simulink model "gm_sampleModel1607_1_sub"  (R2023a)
settings: Solver=VariableStepAuto  StartTime=0.0  StopTime=10.0  RelTol=1e-3
libraries: simulink x1, hdlsllib x1
settings Model: Creator=user1  LastModifiedBy=user1
settings OptimizationCC: BlockReduction=off  ConditionallyExecuteInputs=off
settings DebuggingCC: InheritedTsInSrcMsg=none

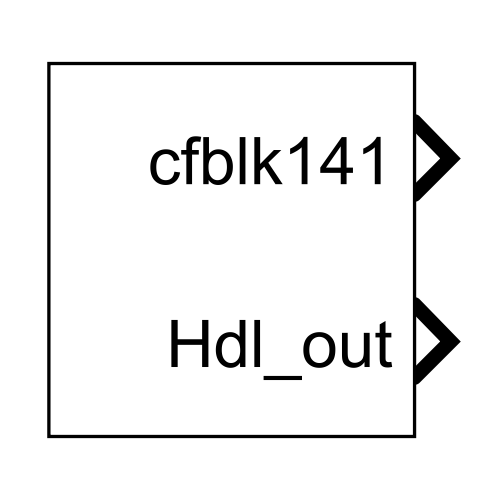
[thumbnail: Simulink's stored preview of the top-level diagram]
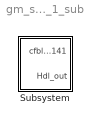
== system gm_sampleModel1607_1_sub ==
  Subsystem : Subsystem

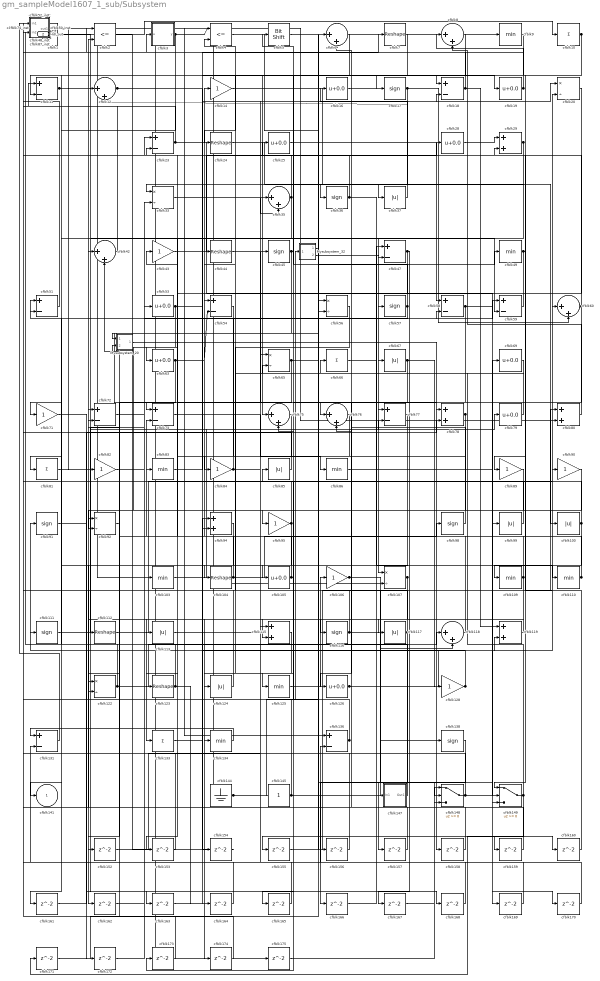
== system gm_sampleModel1607_1_sub/Subsystem ==
  Mysubsystem_20 : Subsystem
  Mysubsystem_32 : Subsystem
  cfblk1 : simulink/Logic and Bit Operations/Extract Bits  bitsToExtract=Upper half  numBits=8  bitIdxRange=[0 7]  outScalingMode=Preserve fixed-point scaling
      settings: LibrarySourceBlock=|
      | hdlsllib/Logic and Bit
      | Operations/Extract Bits
  cfblk{10,66,81,133} (4 alike) : Sum  Inputs=+  OutDataTypeStr=uint8
  cfblk{37,67,85,99..100,113,117,124} (8 alike) : Abs  OutDataTypeStr=uint8  SaturateOnIntegerOverflow=off
  cfblk101_inst : Subsystem
  cfblk{9,49,83,86,103,109..110,125,134} (9 alike) : MinMax  OutDataTypeStr=uint8
  cfblk{7,24,44,104,112,123} (6 alike) : Reshape
  cfblk{16,19,25,28,53,63,69,79,105,126} (10 alike) : Bias  Bias=0.0  SaturateOnIntegerOverflow=off
  cfblk{14,43,71,82,84,89..90,95,106,128} (10 alike) : Gain  OutDataTypeStr=uint8
  cfblk{20,33,56,65,92,107,122} (7 alike) : Product  Inputs=*/  OutDataTypeStr=uint8  RndMeth=Zero  SaturateOnIntegerOverflow=on
  cfblk{11,18,23,47,51,54,58..59,72..73,77,131,136} (13 alike) : Sum  Inputs=+-  OutDataTypeStr=uint8
  cfblk{17,36,45,57,91,98,111,116,138} (9 alike) : Signum
  cfblk{29,78,80,94,115,119} (6 alike) : Sum  OutDataTypeStr=uint8
  cfblk{6,8,12,35,42,60,75..76,118} (9 alike) : Sum  Inputs=|++  OutDataTypeStr=uint8
  cfblk130_inst : Subsystem
  cfblk144 : Ground
  cfblk145 : Constant  OutDataTypeStr=uint8  SampleTime=-1
  cfblk147 : Subsystem
  cfblk148 : Switch  OutDataTypeStr=uint8  SaturateOnIntegerOverflow=off  InputSameDT=off
  cfblk149 : Switch  OutDataTypeStr=uint8  SaturateOnIntegerOverflow=off  InputSameDT=off
  cfblk{152..175} (24 alike) : Delay  SampleTime=1
  cfblk15_inst : Subsystem
  cfblk2 : RelationalOperator  Operator=<=  OutDataTypeStr=boolean  InputSameDT=off
  cfblk3 : Subsystem  mask(Compare To Zero){relop=<=, OutDataTypeStr=uint8, ZeroCross=on}
      mask prompts: relop "Simulink:masks:Operator_MP"; OutDataTypeStr "Simulink:masks:OutputDataType_MP"; ZeroCross "Simulink:masks:EnableZerocrossingDetection_MP"
      mask help: Simulink:masks:CompareToZero_MD
      mask init:
      | OutDataTypeStr = 'uint8';
      | ZeroCross = 'on';
      | blkName = 'sampleModel1607_1_sub/Subsystem/cfblk3';
      | relop = '<=';
      | setValue = 'fixdt(0, 8)';
      mask TypeOptions relop: == | ~= | < | <= | >= | >
      mask TypeOptions OutDataTypeStr: Simulink:masks:uint8 | Simulink:masks:boolean
      mask Callback ZeroCross: sl('zeroCrossEnable', gcbh);
      mask Display: disp([relop,' 0'])
  cfblk4 : RelationalOperator  Operator=<=  OutDataTypeStr=boolean  InputSameDT=off
  cfblk48_inst : Subsystem
  cfblk5 : hdlsllib/Logic and Bit Operations/Bit Shift  mode=Shift Left Logical  N=0
  cfblk50_inst : Subsystem
  cfblk52_inst : Subsystem
  cfblk74_inst : Subsystem
  cfblk87_inst : Subsystem
  cfblk141 : Outport  OutDataTypeStr=uint8  SampleTime=1  VectorParamsAs1DForOutWhenUnconnected=off
  Hdl_out : Outport  Port=2  OutDataTypeStr=uint8  SampleTime=1
  wires:
  Mysubsystem_20/1(Out1) -> cfblk158/1
  Mysubsystem_32/1(Out1) -> cfblk73/1
  Mysubsystem_32/2(Out2) -> cfblk107/1
  cfblk1/1 -> cfblk59/2
  cfblk10/1 -> cfblk75/1, cfblk149/1
  cfblk100/1 -> cfblk23/2, cfblk109/1
  cfblk101_inst/1(out1) -> cfblk175/1
  cfblk103/1 -> cfblk77/2
  cfblk104/1 -> cfblk98/1, cfblk73/2
  cfblk105/1 -> cfblk173/1, cfblk14/1
  cfblk106/1 -> cfblk138/1, cfblk118/2
  cfblk107/1 -> cfblk174/1, cfblk133/1
  cfblk109/1 -> cfblk43/1, cfblk162/1
  cfblk11/1 -> cfblk47/2, cfblk168/1
  cfblk110/1 -> cfblk54/1, cfblk83/1
  cfblk111/1 -> cfblk79/1
  cfblk112/1 -> cfblk69/1
  cfblk113/1 -> cfblk45/1
  cfblk115/1 -> cfblk134/1
  cfblk116/1 -> cfblk2/2, cfblk149/3
  cfblk117/1 -> cfblk4/2, cfblk157/1
  cfblk118/1 -> Mysubsystem_20/2(In2)
  cfblk119/1 -> cfblk115/2
  cfblk12/1 -> cfblk18/1, cfblk154/1
  cfblk122/1 -> cfblk50_inst/2(in2), cfblk118/1
  cfblk123/1 -> cfblk91/1, cfblk164/1
  cfblk124/1 -> cfblk48_inst/2(in2)
  cfblk125/1 -> cfblk106/1
  cfblk126/1 -> cfblk99/1, cfblk20/2
  cfblk128/1 -> cfblk6/2, cfblk111/1
  cfblk130_inst/1(out1) -> cfblk17/1
  cfblk131/1 -> cfblk52_inst/1(in1)
  cfblk133/1 -> cfblk94/1
  cfblk134/1 -> cfblk131/1
  cfblk136/1 -> cfblk85/1, cfblk72/1
  cfblk138/1 -> cfblk166/1
  cfblk14/1 -> cfblk37/1
  cfblk144/1 -> cfblk6/1, Mysubsystem_32/1(In1)
  cfblk145/1 -> cfblk60/1, cfblk149/2, cfblk101_inst/2(in2)
  cfblk147/1(Out1) -> cfblk51/1
  cfblk148/1 -> cfblk52_inst/2(in2), cfblk90/1
  cfblk149/1 -> cfblk171/1, cfblk66/1
  cfblk15_inst/1(out1) -> cfblk107/2, cfblk147/1(In1)
  cfblk152/1 -> cfblk35/1
  cfblk153/1 -> cfblk50_inst/1(in1)
  cfblk154/1 -> cfblk1/1
  cfblk155/1 -> cfblk80/1
  cfblk156/1 -> cfblk42/2
  cfblk157/1 -> cfblk122/2
  cfblk158/1 -> cfblk74_inst/1(in1)
  cfblk159/1 -> cfblk76/2
  cfblk16/1 -> cfblk19/1
  cfblk160/1 -> cfblk29/2
  cfblk161/1 -> cfblk78/2
  cfblk162/1 -> cfblk33/2
  cfblk163/1 -> cfblk119/2
  cfblk164/1 -> cfblk131/2
  cfblk165/1 -> cfblk115/1
  cfblk166/1 -> cfblk47/1
  cfblk167/1 -> cfblk148/3
  cfblk168/1 -> cfblk15_inst/1(in1)
  cfblk169/1 -> cfblk136/2
  cfblk17/1 -> cfblk60/2, cfblk12/2, cfblk33/1
  cfblk170/1 -> cfblk87_inst/1(in1)
  cfblk171/1 -> cfblk56/2
  cfblk172/1 -> cfblk59/1
  cfblk173/1 -> cfblk72/2
  cfblk174/1 -> cfblk130_inst/2(in2)
  cfblk175/1 -> cfblk148/1
  cfblk18/1 -> cfblk87_inst/2(in2), cfblk119/1
  cfblk19/1 -> cfblk8/1, cfblk11/2, cfblk3/1(u)
  cfblk2/1 -> cfblk10/1
  cfblk20/1 -> cfblk105/1
  cfblk23/1 -> cfblk11/1, cfblk169/1
  cfblk24/1 -> cfblk100/1
  cfblk25/1 -> cfblk58/1
  cfblk28/1 -> cfblk29/1
  cfblk29/1 -> cfblk36/1, cfblk161/1
  cfblk3/1(y) -> cfblk4/1, cfblk71/1
  cfblk33/1 -> cfblk35/2
  cfblk35/1 -> cfblk63/1, cfblk15_inst/2(in2)
  cfblk36/1 -> cfblk25/1, cfblk110/1
  cfblk37/1 -> cfblk16/1
  cfblk4/1 -> cfblk156/1
  cfblk42/1 -> cfblk130_inst/1(in1)
  cfblk43/1 -> cfblk28/1
  cfblk44/1 -> cfblk77/1
  cfblk45/1 -> cfblk159/1, Mysubsystem_20/1(In1)
  cfblk47/1 -> cfblk67/1, cfblk123/1, cfblk167/1
  cfblk48_inst/1(out1) -> Hdl_out/1, cfblk103/1
  cfblk49/1 -> cfblk117/1, cfblk89/1
  cfblk5/1 -> cfblk148/2
  cfblk50_inst/1(out1) -> cfblk136/1
  cfblk51/1 -> cfblk74_inst/2(in2)
  cfblk52_inst/1(out1) -> cfblk80/2
  cfblk53/1 -> cfblk92/2, cfblk20/1
  cfblk54/1 -> cfblk153/1
  cfblk56/1 -> cfblk104/1
  cfblk57/1 -> cfblk51/2, cfblk5/1
  cfblk58/1 -> cfblk76/1, cfblk160/1
  cfblk59/1 -> cfblk57/1
  cfblk6/1 -> cfblk165/1
  cfblk60/1 -> cfblk23/1, cfblk126/1
  cfblk63/1 -> cfblk54/2, cfblk92/1
  cfblk65/1 -> cfblk113/1, cfblk49/1
  cfblk66/1 -> cfblk58/2
  cfblk67/1 -> cfblk128/1, cfblk125/1
  cfblk69/1 -> cfblk65/2
  cfblk7/1 -> cfblk75/2
  cfblk71/1 -> cfblk172/1
  cfblk72/1 -> cfblk78/1
  cfblk73/1 -> cfblk86/1
  cfblk74_inst/1(out1) -> cfblk12/1
  cfblk75/1 -> cfblk124/1
  cfblk76/1 -> cfblk94/2
  cfblk77/1 -> cfblk155/1
  cfblk78/1 -> cfblk116/1, cfblk84/1
  cfblk79/1 -> cfblk44/1
  cfblk8/1 -> cfblk24/1
  cfblk80/1 -> cfblk8/2
  cfblk81/1 -> cfblk53/1
  cfblk82/1 -> cfblk56/1
  cfblk83/1 -> cfblk7/1
  cfblk84/1 -> cfblk42/1, cfblk18/2
  cfblk85/1 -> cfblk101_inst/1(in1)
  cfblk86/1 -> cfblk170/1
  cfblk87_inst/1(out1) -> cfblk82/1, cfblk9/1
  cfblk89/1 -> cfblk95/1
  cfblk9/1 -> cfblk81/1
  cfblk90/1 -> cfblk122/1
  cfblk91/1 -> cfblk163/1
  cfblk92/1 -> cfblk152/1
  cfblk94/1 -> cfblk112/1
  cfblk95/1 -> cfblk48_inst/1(in1), cfblk141/1
  cfblk98/1 -> cfblk2/1
  cfblk99/1 -> cfblk65/1

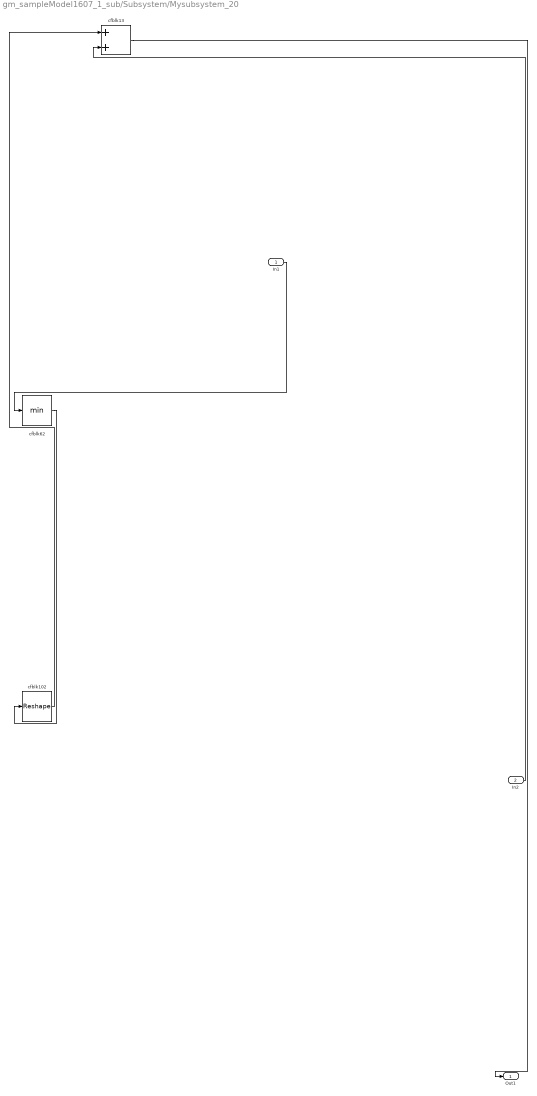
== system gm_sampleModel1607_1_sub/Subsystem/Mysubsystem_20 ==
  In1 : Inport  OutDataTypeStr=uint8  PortDimensions=1  SampleTime=1
  In2 : Inport  Port=2  OutDataTypeStr=uint8  PortDimensions=1  SampleTime=1
  cfblk102 : Reshape
  cfblk13 : Sum
  cfblk62 : MinMax
  Out1 : Outport  SampleTime=1
  wires:
  In1/1 -> cfblk62/1
  In2/1 -> cfblk13/2
  cfblk102/1 -> cfblk13/1
  cfblk13/1 -> Out1/1
  cfblk62/1 -> cfblk102/1

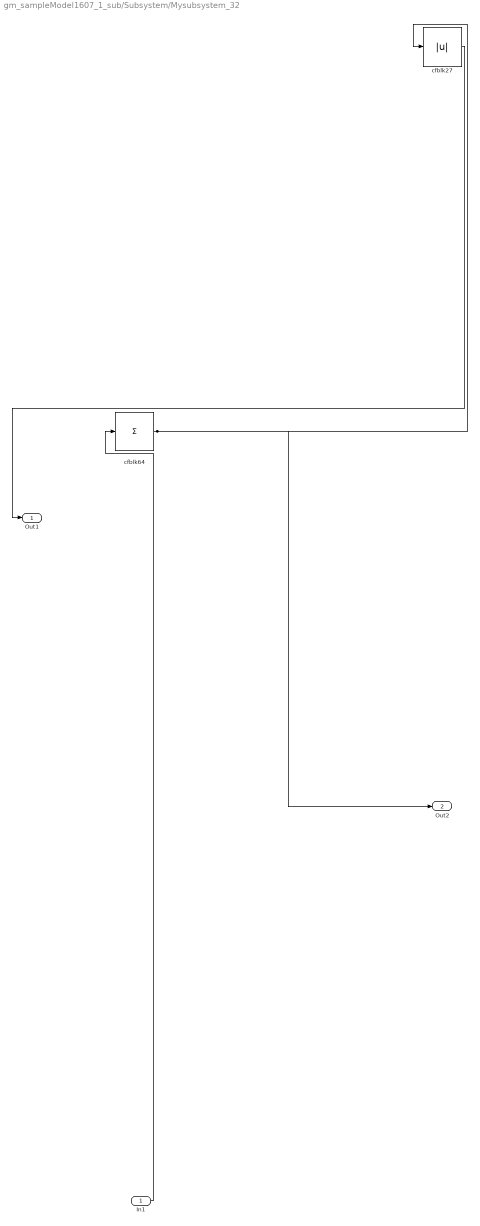
== system gm_sampleModel1607_1_sub/Subsystem/Mysubsystem_32 ==
  In1 : Inport  OutDataTypeStr=uint8  PortDimensions=1  SampleTime=1
  cfblk27 : Abs  SaturateOnIntegerOverflow=off
  cfblk64 : Sum  Inputs=+
  Out1 : Outport  SampleTime=1
  Out2 : Outport  Port=2  SampleTime=1
  wires:
  In1/1 -> cfblk64/1
  cfblk27/1 -> Out1/1
  cfblk64/1 -> cfblk27/1, Out2/1

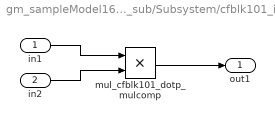
== system gm_sampleModel1607_1_sub/Subsystem/cfblk101_inst ==
  in1 : Inport  OutDataTypeStr=uint8  SampleTime=1
  in2 : Inport  Port=2  OutDataTypeStr=uint8  SampleTime=1
  mul_cfblk101_dotp_mulcomp : Product  Inputs=**  OutDataTypeStr=uint8  SampleTime=1
  out1 : Outport  OutDataTypeStr=uint8  SampleTime=1
  wires:
  in1/1 -> mul_cfblk101_dotp_mulcomp/1
  in2/1 -> mul_cfblk101_dotp_mulcomp/2
  mul_cfblk101_dotp_mulcomp/1 -> out1/1

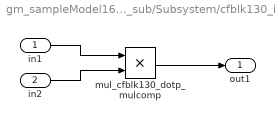
== system gm_sampleModel1607_1_sub/Subsystem/cfblk130_inst ==
  in1 : Inport  OutDataTypeStr=uint8  SampleTime=1
  in2 : Inport  Port=2  OutDataTypeStr=uint8  SampleTime=1
  mul_cfblk130_dotp_mulcomp : Product  Inputs=**  OutDataTypeStr=uint8  SampleTime=1
  out1 : Outport  OutDataTypeStr=uint8  SampleTime=1
  wires:
  in1/1 -> mul_cfblk130_dotp_mulcomp/1
  in2/1 -> mul_cfblk130_dotp_mulcomp/2
  mul_cfblk130_dotp_mulcomp/1 -> out1/1

== system gm_sampleModel1607_1_sub/Subsystem/cfblk147 ==
  In1 : Inport  OutDataTypeStr=uint8  PortDimensions=1  SampleTime=1
  Out1 : Outport  SampleTime=1
  wires:
  In1/1 -> Out1/1

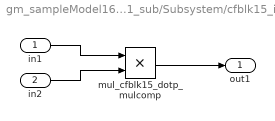
== system gm_sampleModel1607_1_sub/Subsystem/cfblk15_inst ==
  in1 : Inport  OutDataTypeStr=uint8  SampleTime=1
  in2 : Inport  Port=2  OutDataTypeStr=uint8  SampleTime=1
  mul_cfblk15_dotp_mulcomp : Product  Inputs=**  OutDataTypeStr=uint8  SampleTime=1
  out1 : Outport  OutDataTypeStr=uint8  SampleTime=1
  wires:
  in1/1 -> mul_cfblk15_dotp_mulcomp/1
  in2/1 -> mul_cfblk15_dotp_mulcomp/2
  mul_cfblk15_dotp_mulcomp/1 -> out1/1

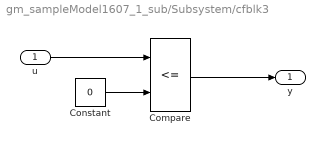
== system gm_sampleModel1607_1_sub/Subsystem/cfblk3 ==
  u : Inport  OutDataTypeStr=uint8  SampleTime=1
  Compare : RelationalOperator  Operator=<=  OutDataTypeStr=fixdt(0, 8)
  Constant : Constant  DisableCoverage=on  Value=0  OutDataTypeStr=Inherit: Inherit via back propagation  SampleTime=-1  PreserveConstantTs=on
  y : Outport  SampleTime=1
  wires:
  u/1 -> Compare/1
  Compare/1 -> y/1
  Constant/1 -> Compare/2

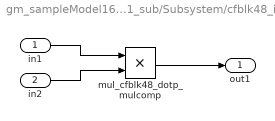
== system gm_sampleModel1607_1_sub/Subsystem/cfblk48_inst ==
  in1 : Inport  OutDataTypeStr=uint8  SampleTime=1
  in2 : Inport  Port=2  OutDataTypeStr=uint8  SampleTime=1
  mul_cfblk48_dotp_mulcomp : Product  Inputs=**  OutDataTypeStr=uint8  SampleTime=1
  out1 : Outport  OutDataTypeStr=uint8  SampleTime=1
  wires:
  in1/1 -> mul_cfblk48_dotp_mulcomp/1
  in2/1 -> mul_cfblk48_dotp_mulcomp/2
  mul_cfblk48_dotp_mulcomp/1 -> out1/1

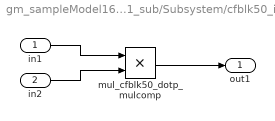
== system gm_sampleModel1607_1_sub/Subsystem/cfblk50_inst ==
  in1 : Inport  OutDataTypeStr=uint8  SampleTime=1
  in2 : Inport  Port=2  OutDataTypeStr=uint8  SampleTime=1
  mul_cfblk50_dotp_mulcomp : Product  Inputs=**  OutDataTypeStr=uint8  SampleTime=1
  out1 : Outport  OutDataTypeStr=uint8  SampleTime=1
  wires:
  in1/1 -> mul_cfblk50_dotp_mulcomp/1
  in2/1 -> mul_cfblk50_dotp_mulcomp/2
  mul_cfblk50_dotp_mulcomp/1 -> out1/1

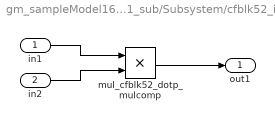
== system gm_sampleModel1607_1_sub/Subsystem/cfblk52_inst ==
  in1 : Inport  OutDataTypeStr=uint8  SampleTime=1
  in2 : Inport  Port=2  OutDataTypeStr=uint8  SampleTime=1
  mul_cfblk52_dotp_mulcomp : Product  Inputs=**  OutDataTypeStr=uint8  SampleTime=1
  out1 : Outport  OutDataTypeStr=uint8  SampleTime=1
  wires:
  in1/1 -> mul_cfblk52_dotp_mulcomp/1
  in2/1 -> mul_cfblk52_dotp_mulcomp/2
  mul_cfblk52_dotp_mulcomp/1 -> out1/1

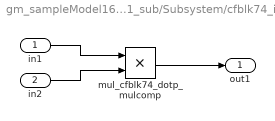
== system gm_sampleModel1607_1_sub/Subsystem/cfblk74_inst ==
  in1 : Inport  OutDataTypeStr=uint8  SampleTime=1
  in2 : Inport  Port=2  OutDataTypeStr=uint8  SampleTime=1
  mul_cfblk74_dotp_mulcomp : Product  Inputs=**  OutDataTypeStr=uint8  SampleTime=1
  out1 : Outport  OutDataTypeStr=uint8  SampleTime=1
  wires:
  in1/1 -> mul_cfblk74_dotp_mulcomp/1
  in2/1 -> mul_cfblk74_dotp_mulcomp/2
  mul_cfblk74_dotp_mulcomp/1 -> out1/1

== system gm_sampleModel1607_1_sub/Subsystem/cfblk87_inst ==
  in1 : Inport  OutDataTypeStr=uint8  SampleTime=1
  in2 : Inport  Port=2  OutDataTypeStr=uint8  SampleTime=1
  mul_cfblk87_dotp_mulcomp : Product  Inputs=**  OutDataTypeStr=uint8  SampleTime=1
  out1 : Outport  OutDataTypeStr=uint8  SampleTime=1
  wires:
  in1/1 -> mul_cfblk87_dotp_mulcomp/1
  in2/1 -> mul_cfblk87_dotp_mulcomp/2
  mul_cfblk87_dotp_mulcomp/1 -> out1/1
